simulink model "CalculDistance"  (R2021b)
settings: Solver=VariableStepAuto  StartTime=0.0  StopTime=10.0  RelTol=1e-3
settings Model: DataDictionary=GuidanceDD.sldd  Creator=Paul  LastModifiedBy=Paul

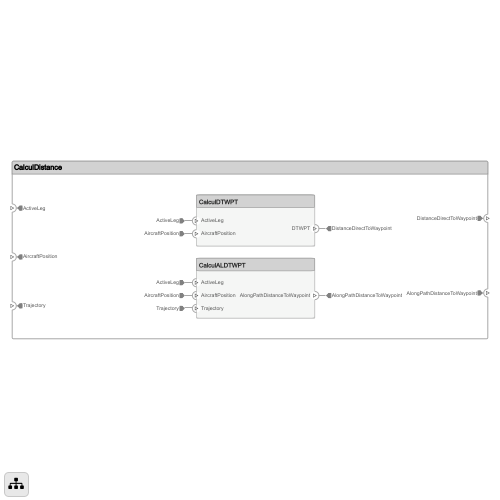
[thumbnail: Simulink's stored preview of the top-level diagram]
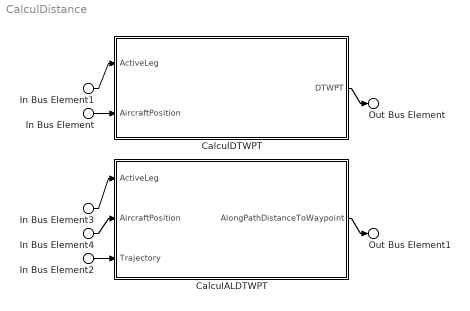
== system CalculDistance ==
  In Bus Element1 : Inport  PortName=ActiveLeg
  In Bus Element3 : Inport  PortName=ActiveLeg
  In Bus Element : Inport  Port=2  PortName=AircraftPosition
  In Bus Element4 : Inport  Port=2  PortName=AircraftPosition
  In Bus Element2 : Inport  Port=3  PortName=Trajectory
  CalculALDTWPT : Subsystem
      settings: PortSchema="{\"entries\":[{\"content\":{\"headerSize\":26,\"margin\":15,\"minimumSpacing\":25,\"sides\":[{\"content\":{\"connectorIds\":[\"In1\",\"In2\",\"In3\"]},\"type\":\"ConnectorPlacement.EquallySpacedRectSide\",\"uuid\":\"6b59cfd3-505c-41dc-bf6c-4d82d451ef5d\"},{\"content\":{\"connectorIds\":[\"Out1\"],\"side\":\"RIGHT\"},\"type\":\"ConnectorPlacement.EquallySpacedRectSide\",\"uuid\":\"f4142fc0-d8fd-40a0-bb01-f33d326facd2\"},{\"content\":{\"connectorIds\":[],\"side\":\"TOP\"},\"type\":\"ConnectorPlacement.EquallySpacedRectSide\",\"uuid\":\"178b855e-eaa2-4b70-a303-d3b7cb6a6ca3\"}]},\"type\":\"ConnectorPlacement.EquallySpacedConnector\",\"uuid\":\"50b576dd-2caa-4080-ba3f-9fa55a69b61e\"}],\"packageUris\":[\"http://schema.mathworks.com/mf0/Connector/R2020b\"],\"version\":\"1.0\"}"
  CalculDTWPT : Subsystem
      settings: PortSchema="{\"entries\":[{\"content\":{\"headerSize\":26,\"margin\":15,\"minimumSpacing\":25,\"sides\":[{\"content\":{\"connectorIds\":[\"In1\",\"In2\"]},\"type\":\"ConnectorPlacement.EquallySpacedRectSide\",\"uuid\":\"6b59cfd3-505c-41dc-bf6c-4d82d451ef5d\"},{\"content\":{\"connectorIds\":[\"Out1\"],\"side\":\"RIGHT\"},\"type\":\"ConnectorPlacement.EquallySpacedRectSide\",\"uuid\":\"f4142fc0-d8fd-40a0-bb01-f33d326facd2\"},{\"content\":{\"connectorIds\":[],\"side\":\"TOP\"},\"type\":\"ConnectorPlacement.EquallySpacedRectSide\",\"uuid\":\"178b855e-eaa2-4b70-a303-d3b7cb6a6ca3\"}]},\"type\":\"ConnectorPlacement.EquallySpacedConnector\",\"uuid\":\"50b576dd-2caa-4080-ba3f-9fa55a69b61e\"}],\"packageUris\":[\"http://schema.mathworks.com/mf0/Connector/R2020b\"],\"version\":\"1.0\"}"
  Out Bus Element : Outport  PortName=DistanceDirectToWaypoint
  Out Bus Element1 : Outport  Port=2  PortName=AlongPathDistanceToWaypoint
  wires:
  In Bus Element1/1 -> CalculDTWPT/1(ActiveLeg)
  In Bus Element/1 -> CalculDTWPT/2(AircraftPosition)
  In Bus Element2/1 -> CalculALDTWPT/3(Trajectory)
  CalculDTWPT/1(DTWPT) -> Out Bus Element/1
  CalculALDTWPT/1(AlongPathDistanceToWaypoint) -> Out Bus Element1/1
  In Bus Element3/1 -> CalculALDTWPT/1(ActiveLeg)
  In Bus Element4/1 -> CalculALDTWPT/2(AircraftPosition)

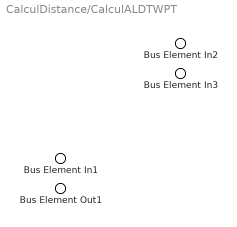
== system CalculDistance/CalculALDTWPT ==
  Bus Element In3 : Inport  PortName=ActiveLeg
  Bus Element In2 : Inport  Port=2  PortName=AircraftPosition
  Bus Element In1 : Inport  Port=3  PortName=Trajectory
  Bus Element Out1 : Outport  PortName=AlongPathDistanceToWaypoint

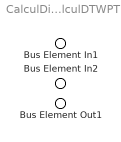
== system CalculDistance/CalculDTWPT ==
  Bus Element In1 : Inport  PortName=ActiveLeg
  Bus Element In2 : Inport  Port=2  PortName=AircraftPosition
  Bus Element Out1 : Outport  PortName=DTWPT
